simulink library "ntbdc"  (Simulink 8.1)
settings: Solver=ode1  StartTime=0.0  StopTime=Inf  FixedStep=0.001  RelTol=1e-3
PostLoadFcn:
  | , if any(exist('dsrtsu_mdlpostloadfcn', 'file') == [2, 3, 6]), try dsrtsu_mdlpostloadfcn('Execute', bdroot); catch fprintf('Error in PostLoadFcn (dsrtsu_mdlpostloadfcn) for model "%s":\n %s\n', bdroot, lasterr); end, end,
settings Model: DSRTSU_INTERNAL_RTI_VER=450  DSRTSU_INTERNAL_RTI_TYPE=rti1401  Creator=tescamilla  LastModifiedBy=tescamilla

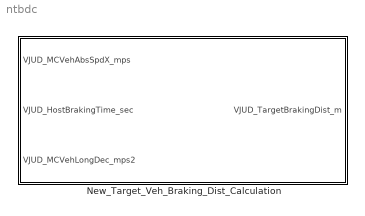
== system ntbdc ==
  New_Target_Veh_Braking_Dist_Calculation : Subsystem

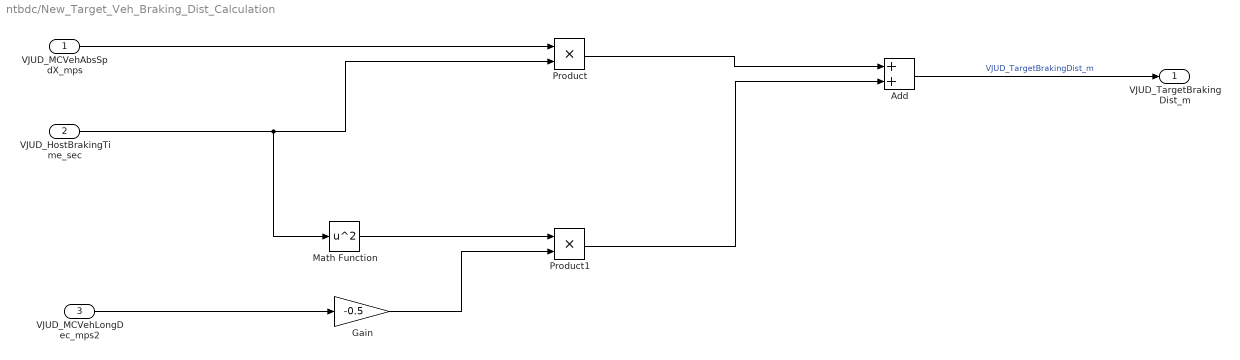
== system ntbdc/New_Target_Veh_Braking_Dist_Calculation ==
  VJUD_MCVehAbsSpdX_mps : Inport
  VJUD_HostBrakingTime_sec : Inport  Port=2
  VJUD_MCVehLongDec_mps2 : Inport  Port=3
  Add : Sum
  Gain : Gain  Gain=-0.5  OutDataTypeStr=single
  Math Function : Math  Operator=square  SaturateOnIntegerOverflow=on
  Product : Product
  Product1 : Product
  VJUD_TargetBrakingDist_m : Outport
  wires:
  Add/1 -> VJUD_TargetBrakingDist_m/1  "VJUD_TargetBrakingDist_m"
  VJUD_MCVehAbsSpdX_mps/1 -> Product/1
  VJUD_HostBrakingTime_sec/1 -> Math Function/1, Product/2
  Math Function/1 -> Product1/1
  VJUD_MCVehLongDec_mps2/1 -> Gain/1
  Gain/1 -> Product1/2
  Product/1 -> Add/1
  Product1/1 -> Add/2
